simulink model "ES2_4_simulink"  (R2023b)
settings: Solver=VariableStepAuto  StartTime=0.0  StopTime=30.0  RelTol=1e-3
undefined symbols (not defined in the file): fdesignblkfcn, gcbh
libraries: dspfdesign x4, dspstat3 x4, simulink x4, vrlib x2
settings Model: NumberOfSteps=100  Creator=manu  LastModifiedBy=manu

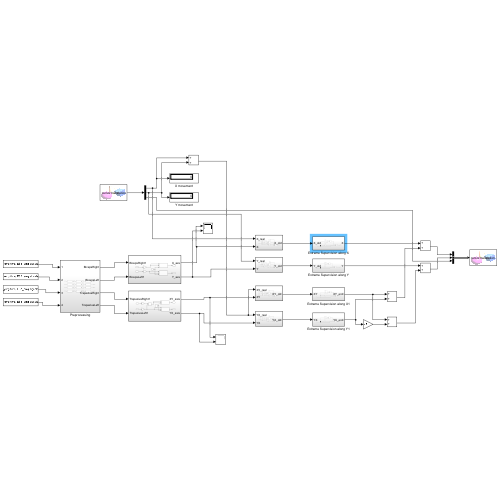
[thumbnail: Simulink's stored preview of the top-level diagram]
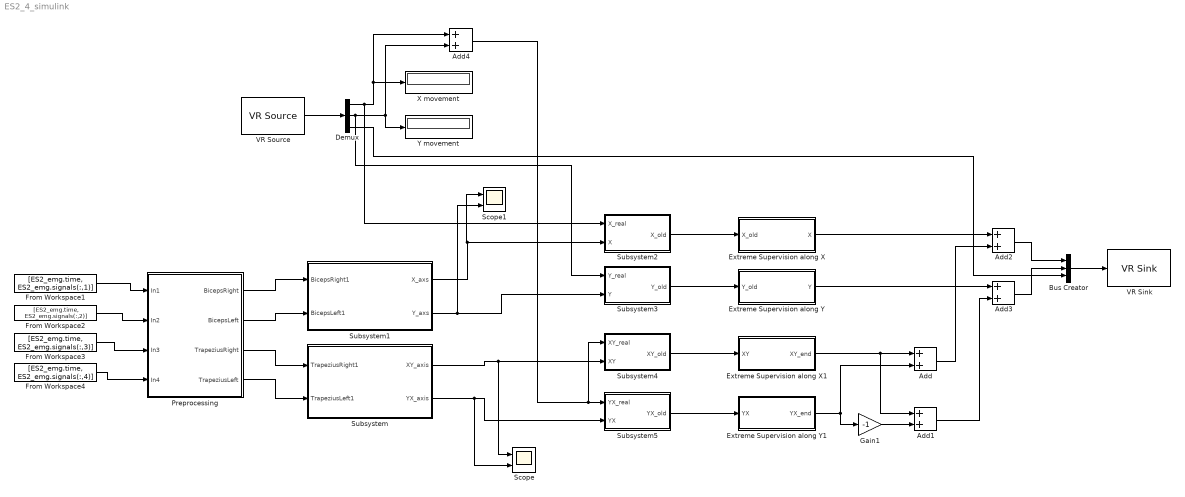
== system ES2_4_simulink ==
  Add{,1..4} (5 alike) : Sum
  Bus Creator : BusCreator  Inputs=3
  Demux : Demux  Outputs=3
  Extreme Supervision along X : Subsystem
  Extreme Supervision along X1 : Subsystem
  Extreme Supervision along Y : Subsystem
  Extreme Supervision along Y1 : Subsystem
  From Workspace1 : FromWorkspace  VariableName=[ES2_emg.time, ES2_emg.signals(:,1)]  OutDataTypeStr=double  SampleTime=0.001
  From Workspace2 : FromWorkspace  VariableName=[ES2_emg.time, ES2_emg.signals(:,2)]  OutDataTypeStr=double  SampleTime=0.001
  From Workspace3 : FromWorkspace  VariableName=[ES2_emg.time, ES2_emg.signals(:,3)]  OutDataTypeStr=double  SampleTime=0.001
  From Workspace4 : FromWorkspace  VariableName=[ES2_emg.time, ES2_emg.signals(:,4)]  OutDataTypeStr=double  SampleTime=0.001
  Gain1 : Gain  Gain=-1
  Preprocessing : Subsystem
  Scope : Scope  NumInputPorts=2
  Scope1 : Scope  NumInputPorts=2
  Subsystem : Subsystem
  Subsystem1 : Subsystem
  Subsystem2 : Subsystem
  Subsystem3 : Subsystem
  Subsystem4 : Subsystem
  Subsystem5 : Subsystem
  VR Sink : vrlib/VR Sink  InstantiateOnLoad=on  SampleTime=0.1  ViewEnable=on  RemoteChange=off  RemoteView=off  FieldsWritten=cursor.translation.3.1.1.double  WorldFileName=8_palline_color.wrl  AutoView=off  VideoDimensions=[]  AllowVariableSize=off
  VR Source : vrlib/VR Source  InstantiateOnLoad=on  SampleTime=0.1  ViewEnable=on  RemoteChange=off  RemoteView=off  FieldsRead=cursor.translation.1.3.1.double  WorldFileName=8_palline_color.wrl  AutoView=off  VideoDimensions=[]  AllowVariableSize=off
  X movement : Display
  Y movement : Display
  wires:
  From Workspace1/1 -> Preprocessing/1(In1)
  From Workspace2/1 -> Preprocessing/2(In2)
  From Workspace3/1 -> Preprocessing/3(In3)
  From Workspace4/1 -> Preprocessing/4(In4)
  Bus Creator/1 -> VR Sink/1
  VR Source/1 -> Demux/1
  Demux/3 -> Bus Creator/3
  Demux/1 -> Subsystem2/1(X_real), X movement/1, Add4/1
  Demux/2 -> Y movement/1, Add4/2, Subsystem3/1(Y_real)
  Subsystem1/1(X_axs) -> Scope1/1, Subsystem2/2(X)
  Subsystem2/1(X_old) -> Extreme Supervision along X/1(X_old)
  Subsystem1/2(Y_axs) -> Scope1/2, Subsystem3/2(Y)
  Subsystem3/1(Y_old) -> Extreme Supervision along Y/1(Y_old)
  Add/1 -> Add2/2
  Extreme Supervision along X1/1(XY_end) -> Add1/1, Add/1
  Extreme Supervision along Y1/1(YX_end) -> Gain1/1, Add/2
  Gain1/1 -> Add1/2
  Add1/1 -> Add3/2
  Extreme Supervision along X/1(X) -> Add2/1
  Add2/1 -> Bus Creator/1
  Extreme Supervision along Y/1(Y) -> Add3/1
  Add3/1 -> Bus Creator/2
  Subsystem4/1(XY_old) -> Extreme Supervision along X1/1(XY)
  Subsystem5/1(YX_old) -> Extreme Supervision along Y1/1(YX)
  Add4/1 -> Subsystem5/1(YX_real), Subsystem4/1(XY_real)
  Preprocessing/1(BicepsRight) -> Subsystem1/1(BicepsRight1)
  Preprocessing/2(BicepsLeft) -> Subsystem1/2(BicepsLeft1)
  Preprocessing/3(TrapeziusRight) -> Subsystem/1(TrapeziusRight1)
  Preprocessing/4(TrapeziusLeft) -> Subsystem/2(TrapeziusLeft1)
  Subsystem/1(XY_axis) -> Subsystem4/2(XY), Scope/1
  Subsystem/2(YX_axis) -> Scope/2, Subsystem5/2(YX)

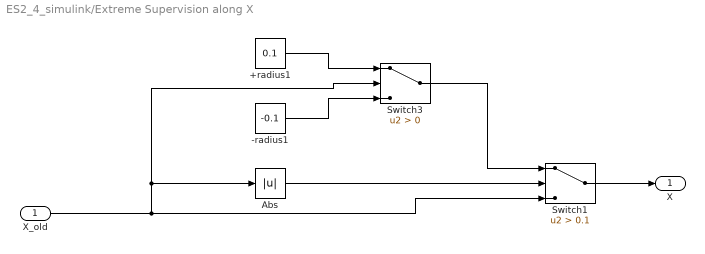
== system ES2_4_simulink/Extreme Supervision along X ==
  X_old : Inport
  +radius1 : Constant  Value=0.1
  -radius1 : Constant  Value=-0.1
  Abs : Abs  SaturateOnIntegerOverflow=off
  Switch1 : Switch  Criteria=u2 > Threshold  Threshold=0.1  SaturateOnIntegerOverflow=off  InputSameDT=off
  Switch3 : Switch  Criteria=u2 > Threshold  SaturateOnIntegerOverflow=off  InputSameDT=off
  X : Outport
  wires:
  Switch3/1 -> Switch1/1
  Abs/1 -> Switch1/2
  +radius1/1 -> Switch3/1
  X_old/1 -> Switch3/2, Abs/1, Switch1/3
  -radius1/1 -> Switch3/3
  Switch1/1 -> X/1

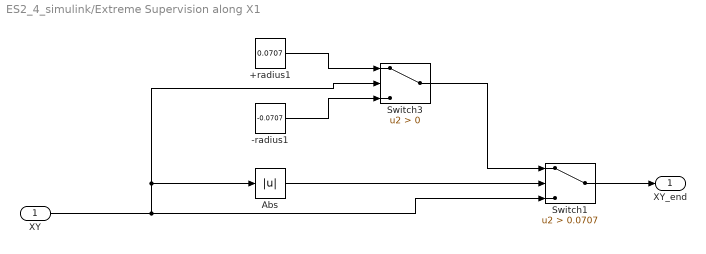
== system ES2_4_simulink/Extreme Supervision along X1 ==
  XY : Inport
  +radius1 : Constant  Value=0.0707
  -radius1 : Constant  Value=-0.0707
  Abs : Abs  SaturateOnIntegerOverflow=off
  Switch1 : Switch  Criteria=u2 > Threshold  Threshold=0.0707  SaturateOnIntegerOverflow=off  InputSameDT=off
  Switch3 : Switch  Criteria=u2 > Threshold  SaturateOnIntegerOverflow=off  InputSameDT=off
  XY_end : Outport
  wires:
  Switch3/1 -> Switch1/1
  Abs/1 -> Switch1/2
  +radius1/1 -> Switch3/1
  XY/1 -> Switch3/2, Abs/1, Switch1/3
  -radius1/1 -> Switch3/3
  Switch1/1 -> XY_end/1

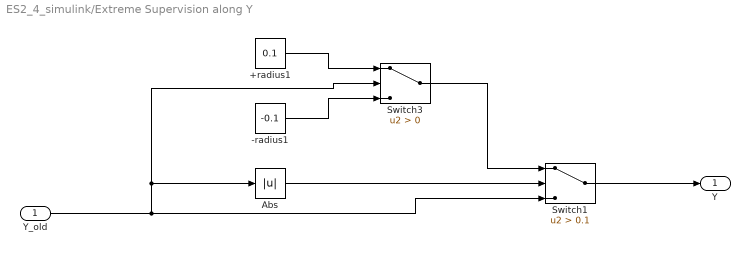
== system ES2_4_simulink/Extreme Supervision along Y ==
  Y_old : Inport
  +radius1 : Constant  Value=0.1
  -radius1 : Constant  Value=-0.1
  Abs : Abs  SaturateOnIntegerOverflow=off
  Switch1 : Switch  Criteria=u2 > Threshold  Threshold=0.1  SaturateOnIntegerOverflow=off  InputSameDT=off
  Switch3 : Switch  Criteria=u2 > Threshold  SaturateOnIntegerOverflow=off  InputSameDT=off
  Y : Outport
  wires:
  Switch3/1 -> Switch1/1
  Abs/1 -> Switch1/2
  +radius1/1 -> Switch3/1
  Y_old/1 -> Switch3/2, Abs/1, Switch1/3
  -radius1/1 -> Switch3/3
  Switch1/1 -> Y/1

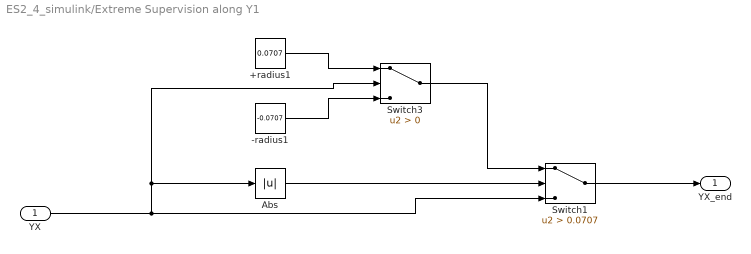
== system ES2_4_simulink/Extreme Supervision along Y1 ==
  YX : Inport
  +radius1 : Constant  Value=0.0707
  -radius1 : Constant  Value=-0.0707
  Abs : Abs  SaturateOnIntegerOverflow=off
  Switch1 : Switch  Criteria=u2 > Threshold  Threshold=0.0707  SaturateOnIntegerOverflow=off  InputSameDT=off
  Switch3 : Switch  Criteria=u2 > Threshold  SaturateOnIntegerOverflow=off  InputSameDT=off
  YX_end : Outport
  wires:
  Switch3/1 -> Switch1/1
  Abs/1 -> Switch1/2
  +radius1/1 -> Switch3/1
  YX/1 -> Switch3/2, Abs/1, Switch1/3
  -radius1/1 -> Switch3/3
  Switch1/1 -> YX_end/1

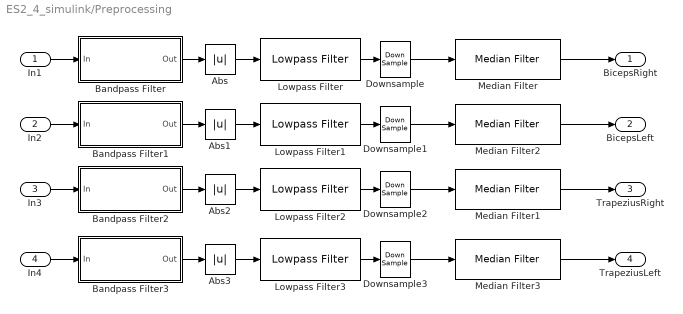
== system ES2_4_simulink/Preprocessing ==
  In1 : Inport
  In2 : Inport  Port=2
  In3 : Inport  Port=3
  In4 : Inport  Port=4
  Abs{,1..3} (4 alike) : Abs  SaturateOnIntegerOverflow=off
  Bandpass Filter : Subsystem  DialogController=fdesignblkfcn  InitFcn=fdesignblkfcn(gcbh, {'InitFcn'});  mask(Bandpass Filter){}
      mask help: dsp:DSPFilterDesignBlockDialog:BandpassFdesign_MaskDesc
      settings: CopyFcn=fdesignblkfcn(gcbh, {'CopyFcn'});
      mask Help: helpview(mapfilelocation('dsp'), 'dspbandpassfilter');
      mask Display: disp('Bandpass');
  Bandpass Filter1 : Subsystem  DialogController=fdesignblkfcn  InitFcn=fdesignblkfcn(gcbh, {'InitFcn'});  mask(Bandpass Filter){}
      mask help: dsp:DSPFilterDesignBlockDialog:BandpassFdesign_MaskDesc
      settings: CopyFcn=fdesignblkfcn(gcbh, {'CopyFcn'});
      mask Help: helpview(mapfilelocation('dsp'), 'dspbandpassfilter');
      mask Display: disp('Bandpass');
  Bandpass Filter2 : Subsystem  DialogController=fdesignblkfcn  InitFcn=fdesignblkfcn(gcbh, {'InitFcn'});  mask(Bandpass Filter){}
      mask help: dsp:DSPFilterDesignBlockDialog:BandpassFdesign_MaskDesc
      settings: CopyFcn=fdesignblkfcn(gcbh, {'CopyFcn'});
      mask Help: helpview(mapfilelocation('dsp'), 'dspbandpassfilter');
      mask Display: disp('Bandpass');
  Bandpass Filter3 : Subsystem  DialogController=fdesignblkfcn  InitFcn=fdesignblkfcn(gcbh, {'InitFcn'});  mask(Bandpass Filter){}
      mask help: dsp:DSPFilterDesignBlockDialog:BandpassFdesign_MaskDesc
      settings: CopyFcn=fdesignblkfcn(gcbh, {'CopyFcn'});
      mask Help: helpview(mapfilelocation('dsp'), 'dspbandpassfilter');
      mask Display: disp('Bandpass');
  Downsample{,1..3} (4 alike) : DownSample  N=4  RateOptions=Allow multirate processing
  Lowpass Filter{,1..3} (4 alike) : dspfdesign/Lowpass Filter  FilterType=FIR  DesignForMinimumOrder=on  FilterOrder=50  PassbandFrequency=3  StopbandFrequency=6  PassbandRipple=0.1  StopbandAttenuation=80  SampleRateMode=Specify on dialog  SampleRate=1000  SimulateUsing=Interpreted execution  roundingMode=Floor  coeffsDataTypeStr=fixdt(1,16)
  Median Filter : dspstat3/Median Filter  WindowLength=250  SimulateUsing=Interpreted execution
      settings: LibrarySourceBlock=|
      | dspfdesign/Median
      | Filter
  Median Filter1 : dspstat3/Median Filter  WindowLength=300  SimulateUsing=Interpreted execution
      settings: LibrarySourceBlock=|
      | dspfdesign/Median
      | Filter
  Median Filter2 : dspstat3/Median Filter  WindowLength=250  SimulateUsing=Interpreted execution
      settings: LibrarySourceBlock=|
      | dspfdesign/Median
      | Filter
  Median Filter3 : dspstat3/Median Filter  WindowLength=250  SimulateUsing=Interpreted execution
      settings: LibrarySourceBlock=|
      | dspfdesign/Median
      | Filter
  BicepsRight : Outport
  BicepsLeft : Outport  Port=2
  TrapeziusRight : Outport  Port=3
  TrapeziusLeft : Outport  Port=4
  wires:
  Lowpass Filter2/1 -> Downsample2/1
  Bandpass Filter2/1(Out) -> Abs2/1
  Abs1/1 -> Lowpass Filter1/1
  Abs3/1 -> Lowpass Filter3/1
  Abs/1 -> Lowpass Filter/1
  Bandpass Filter3/1(Out) -> Abs3/1
  In4/1 -> Bandpass Filter3/1(In)
  In1/1 -> Bandpass Filter/1(In)
  Bandpass Filter/1(Out) -> Abs/1
  Bandpass Filter1/1(Out) -> Abs1/1
  Abs2/1 -> Lowpass Filter2/1
  Lowpass Filter1/1 -> Downsample1/1
  Lowpass Filter3/1 -> Downsample3/1
  Lowpass Filter/1 -> Downsample/1
  In3/1 -> Bandpass Filter2/1(In)
  In2/1 -> Bandpass Filter1/1(In)
  Downsample/1 -> Median Filter/1
  Downsample1/1 -> Median Filter2/1
  Downsample2/1 -> Median Filter1/1
  Downsample3/1 -> Median Filter3/1
  Median Filter/1 -> BicepsRight/1
  Median Filter2/1 -> BicepsLeft/1
  Median Filter1/1 -> TrapeziusRight/1
  Median Filter3/1 -> TrapeziusLeft/1

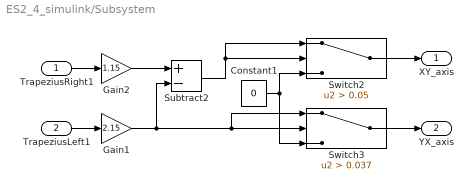
== system ES2_4_simulink/Subsystem ==
  TrapeziusRight1 : Inport
  TrapeziusLeft1 : Inport  Port=2
  Constant1 : Constant  Value=0
  Gain1 : Gain  Gain=2.15
  Gain2 : Gain  Gain=1.15
  Subtract2 : Sum  Inputs=+-
  Switch2 : Switch  Criteria=u2 > Threshold  Threshold=0.05  SaturateOnIntegerOverflow=off  InputSameDT=off
  Switch3 : Switch  Criteria=u2 > Threshold  Threshold=0.037  SaturateOnIntegerOverflow=off  InputSameDT=off
  XY_axis : Outport
  YX_axis : Outport  Port=2
  wires:
  TrapeziusRight1/1 -> Gain2/1
  Constant1/1 -> Switch3/3, Switch2/3
  Gain1/1 -> Subtract2/2, Switch3/1, Switch3/2
  Gain2/1 -> Subtract2/1
  TrapeziusLeft1/1 -> Gain1/1
  Subtract2/1 -> Switch2/1, Switch2/2
  Switch2/1 -> XY_axis/1
  Switch3/1 -> YX_axis/1

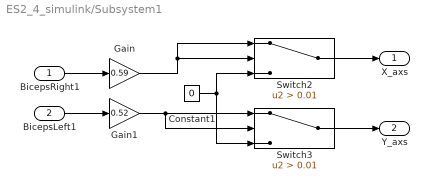
== system ES2_4_simulink/Subsystem1 ==
  BicepsRight1 : Inport
  BicepsLeft1 : Inport  Port=2
  Constant1 : Constant  Value=0
  Gain : Gain  Gain=0.59
  Gain1 : Gain  Gain=0.52
  Switch2 : Switch  Criteria=u2 > Threshold  Threshold=0.01  SaturateOnIntegerOverflow=off  InputSameDT=off
  Switch3 : Switch  Criteria=u2 > Threshold  Threshold=0.01  SaturateOnIntegerOverflow=off  InputSameDT=off
  X_axs : Outport
  Y_axs : Outport  Port=2
  wires:
  BicepsLeft1/1 -> Gain1/1
  BicepsRight1/1 -> Gain/1
  Constant1/1 -> Switch3/3, Switch2/3
  Gain/1 -> Switch2/1, Switch2/2
  Gain1/1 -> Switch3/1, Switch3/2
  Switch2/1 -> X_axs/1
  Switch3/1 -> Y_axs/1

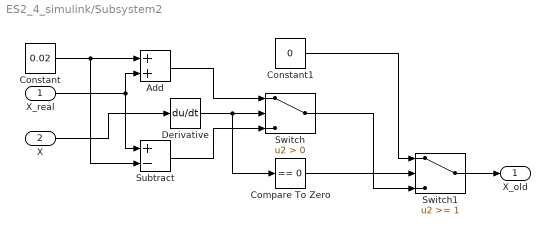
== system ES2_4_simulink/Subsystem2 ==
  X_real : Inport
  X : Inport  Port=2
  Add : Sum
  Compare To Zero : simulink/Logic and Bit Operations/Compare To Zero  relop===  OutDataTypeStr=boolean
  Constant : Constant  Value=0.02
  Constant1 : Constant  Value=0
  Derivative : Derivative
  Subtract : Sum  Inputs=+-
  Switch : Switch  Criteria=u2 > Threshold  SaturateOnIntegerOverflow=off  InputSameDT=off
  Switch1 : Switch  Threshold=1  SaturateOnIntegerOverflow=off  InputSameDT=off
  X_old : Outport
  wires:
  Derivative/1 -> Compare To Zero/1, Switch/2
  Compare To Zero/1 -> Switch1/2
  Constant/1 -> Add/1, Subtract/2
  X_real/1 -> Subtract/1, Add/2
  Constant1/1 -> Switch1/1
  Switch/1 -> Switch1/3
  Add/1 -> Switch/1
  Subtract/1 -> Switch/3
  X/1 -> Derivative/1
  Switch1/1 -> X_old/1

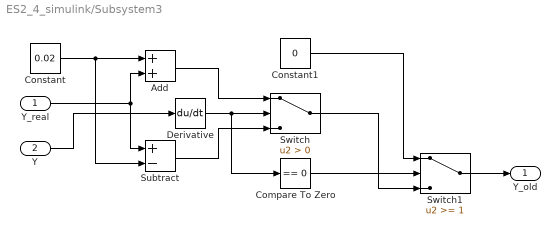
== system ES2_4_simulink/Subsystem3 ==
  Y_real : Inport
  Y : Inport  Port=2
  Add : Sum
  Compare To Zero : simulink/Logic and Bit Operations/Compare To Zero  relop===  OutDataTypeStr=boolean
  Constant : Constant  Value=0.02
  Constant1 : Constant  Value=0
  Derivative : Derivative
  Subtract : Sum  Inputs=+-
  Switch : Switch  Criteria=u2 > Threshold  SaturateOnIntegerOverflow=off  InputSameDT=off
  Switch1 : Switch  Threshold=1  SaturateOnIntegerOverflow=off  InputSameDT=off
  Y_old : Outport
  wires:
  Derivative/1 -> Compare To Zero/1, Switch/2
  Compare To Zero/1 -> Switch1/2
  Constant/1 -> Add/1, Subtract/2
  Y_real/1 -> Add/2, Subtract/1
  Constant1/1 -> Switch1/1
  Switch/1 -> Switch1/3
  Add/1 -> Switch/1
  Subtract/1 -> Switch/3
  Y/1 -> Derivative/1
  Switch1/1 -> Y_old/1

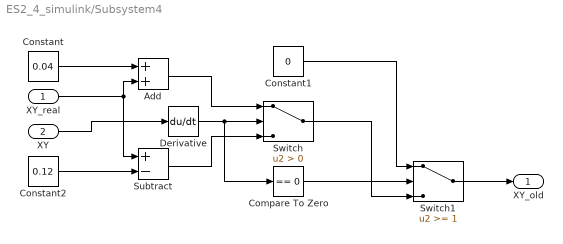
== system ES2_4_simulink/Subsystem4 ==
  XY_real : Inport
  XY : Inport  Port=2
  Add : Sum
  Compare To Zero : simulink/Logic and Bit Operations/Compare To Zero  relop===  OutDataTypeStr=boolean
  Constant : Constant  Value=0.04
  Constant1 : Constant  Value=0
  Constant2 : Constant  Value=0.12
  Derivative : Derivative
  Subtract : Sum  Inputs=+-
  Switch : Switch  Criteria=u2 > Threshold  SaturateOnIntegerOverflow=off  InputSameDT=off
  Switch1 : Switch  Threshold=1  SaturateOnIntegerOverflow=off  InputSameDT=off
  XY_old : Outport
  wires:
  Derivative/1 -> Compare To Zero/1, Switch/2
  Compare To Zero/1 -> Switch1/2
  Constant/1 -> Add/1
  XY_real/1 -> Add/2, Subtract/1
  Constant1/1 -> Switch1/1
  Switch/1 -> Switch1/3
  Add/1 -> Switch/1
  Subtract/1 -> Switch/3
  XY/1 -> Derivative/1
  Switch1/1 -> XY_old/1
  Constant2/1 -> Subtract/2

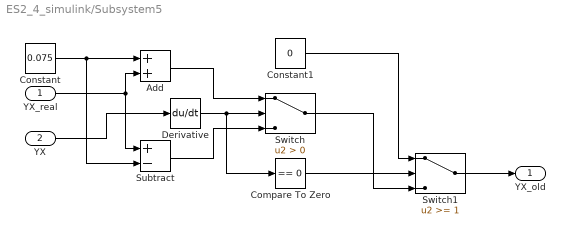
== system ES2_4_simulink/Subsystem5 ==
  YX_real : Inport
  YX : Inport  Port=2
  Add : Sum
  Compare To Zero : simulink/Logic and Bit Operations/Compare To Zero  relop===  OutDataTypeStr=boolean
  Constant : Constant  Value=0.075
  Constant1 : Constant  Value=0
  Derivative : Derivative
  Subtract : Sum  Inputs=+-
  Switch : Switch  Criteria=u2 > Threshold  SaturateOnIntegerOverflow=off  InputSameDT=off
  Switch1 : Switch  Threshold=1  SaturateOnIntegerOverflow=off  InputSameDT=off
  YX_old : Outport
  wires:
  Derivative/1 -> Compare To Zero/1, Switch/2
  Compare To Zero/1 -> Switch1/2
  Constant/1 -> Subtract/2, Add/1
  YX_real/1 -> Subtract/1, Add/2
  Constant1/1 -> Switch1/1
  Switch/1 -> Switch1/3
  Add/1 -> Switch/1
  Subtract/1 -> Switch/3
  YX/1 -> Derivative/1
  Switch1/1 -> YX_old/1

== system ES2_4_simulink/Preprocessing/Bandpass Filter ==
  In : Inport
  Generated Filter Block : DiscreteFir  Tag=BlockMethodSubSystem  Coefficients=[8.09984662039171167e-19 6.39138873735445952e-05 -0.000529985360713195602 0.000163049509978640958 -0.00106873656065133355 0.000138454107623771778 -0.00150740219393306354 -0.000146171169312381939 -0.00164491285071874664 -0.000803831165663842096 -0.00127002939103642264 -0.00179475969145176406 -0.000313202715390952153 -0.00280047053638836797 0.00102378750565708626 -0.00320898606072516192 0.00226847122552957785 -0.00229118992766688115 0.00286273128519679053 0.000444283590646493102 0.00248061645378650983 0.00484772649949967091 0.0013231555973298554 0.00988516690279817554 0.000195375038696813459 0.0137475146561206515 0.000235578061564314939 0.0143783789118079978 0.00232373851233996093 0.0102932854869860792 0.00637980828249819481 0.0013872101835551594 0.0108821641584975915 -0.0106388069047137126 0.0129164407258158982 -0.0225052497171089536 0.00888838159476280226 -0.0302697542973048087 -0.00424164083303872359 -0.0306714306083059364 -0.0276065409272709811 -0.022423923961180349 -0.0594922495550082378 -0.00693651358874992994 -0.0952531612511480497 0.0118816213758879876 -0.128243809353299015 0.0287429432612043914 -0.151547652016043505 0.0386729267839347052 0.839787881504184819 0.0386729267839347052 -0.151547652016043505 0.0287429432612043914 -0.128243809353299015 0.0118816213758879876 -0.0952531612511480497 -0.00693651358874992994 -0.0594922495550082378 -0.022423923961180349 -0.0276065409272709811 -0.0306714306083059364 -0.00424164083303872359 -0.0302697542973048087 0.00888838159476280226 -0.0225052497171089536 0.0129164407258158982 -0.0106388069047137126 0.0108821641584975915 0.0013872101835551594 0.00637980828249819481 0.0102932854869860792 0.00232373851233996093 0.0143783789118079978 0.000235578061564314939 0.0137475146561206515 0.000195375038696813459 0.00988516690279817554 0.0013231555973298554 0.00484772649949967091 0.00248061645378650983 0.000444283590646493102 0.00286273128519679053 -0.00229118992766688115 0.00226847122552957785 -0.00320898606072516192 0.00102378750565708626 -0.00280047053638836797 -0.000313202715390952153 -0.00179475969145176406 -0.00127002939103642264 -0.000803831165663842096 -0.00164491285071874664 -0.000146171169312381939 -0.00150740219393306354 0.000138454107623771778 -0.00106873656065133355 0.000163049509978640958 -0.000529985360713195602 6.39138873735445952e-05 8.09984662039171167e-19]  InputProcessing=Columns as channels (frame based)
  Out : Outport  VectorParamsAs1DForOutWhenUnconnected=off
  wires:
  In/1 -> Generated Filter Block/1
  Generated Filter Block/1 -> Out/1

== system ES2_4_simulink/Preprocessing/Bandpass Filter1 ==
  In : Inport
  Generated Filter Block : DiscreteFir  Tag=BlockMethodSubSystem  Coefficients=[8.09984662039171167e-19 6.39138873735445952e-05 -0.000529985360713195602 0.000163049509978640958 -0.00106873656065133355 0.000138454107623771778 -0.00150740219393306354 -0.000146171169312381939 -0.00164491285071874664 -0.000803831165663842096 -0.00127002939103642264 -0.00179475969145176406 -0.000313202715390952153 -0.00280047053638836797 0.00102378750565708626 -0.00320898606072516192 0.00226847122552957785 -0.00229118992766688115 0.00286273128519679053 0.000444283590646493102 0.00248061645378650983 0.00484772649949967091 0.0013231555973298554 0.00988516690279817554 0.000195375038696813459 0.0137475146561206515 0.000235578061564314939 0.0143783789118079978 0.00232373851233996093 0.0102932854869860792 0.00637980828249819481 0.0013872101835551594 0.0108821641584975915 -0.0106388069047137126 0.0129164407258158982 -0.0225052497171089536 0.00888838159476280226 -0.0302697542973048087 -0.00424164083303872359 -0.0306714306083059364 -0.0276065409272709811 -0.022423923961180349 -0.0594922495550082378 -0.00693651358874992994 -0.0952531612511480497 0.0118816213758879876 -0.128243809353299015 0.0287429432612043914 -0.151547652016043505 0.0386729267839347052 0.839787881504184819 0.0386729267839347052 -0.151547652016043505 0.0287429432612043914 -0.128243809353299015 0.0118816213758879876 -0.0952531612511480497 -0.00693651358874992994 -0.0594922495550082378 -0.022423923961180349 -0.0276065409272709811 -0.0306714306083059364 -0.00424164083303872359 -0.0302697542973048087 0.00888838159476280226 -0.0225052497171089536 0.0129164407258158982 -0.0106388069047137126 0.0108821641584975915 0.0013872101835551594 0.00637980828249819481 0.0102932854869860792 0.00232373851233996093 0.0143783789118079978 0.000235578061564314939 0.0137475146561206515 0.000195375038696813459 0.00988516690279817554 0.0013231555973298554 0.00484772649949967091 0.00248061645378650983 0.000444283590646493102 0.00286273128519679053 -0.00229118992766688115 0.00226847122552957785 -0.00320898606072516192 0.00102378750565708626 -0.00280047053638836797 -0.000313202715390952153 -0.00179475969145176406 -0.00127002939103642264 -0.000803831165663842096 -0.00164491285071874664 -0.000146171169312381939 -0.00150740219393306354 0.000138454107623771778 -0.00106873656065133355 0.000163049509978640958 -0.000529985360713195602 6.39138873735445952e-05 8.09984662039171167e-19]  InputProcessing=Columns as channels (frame based)
  Out : Outport  VectorParamsAs1DForOutWhenUnconnected=off
  wires:
  In/1 -> Generated Filter Block/1
  Generated Filter Block/1 -> Out/1

== system ES2_4_simulink/Preprocessing/Bandpass Filter2 ==
  In : Inport
  Generated Filter Block : DiscreteFir  Tag=BlockMethodSubSystem  Coefficients=[8.09984662039171167e-19 6.39138873735445952e-05 -0.000529985360713195602 0.000163049509978640958 -0.00106873656065133355 0.000138454107623771778 -0.00150740219393306354 -0.000146171169312381939 -0.00164491285071874664 -0.000803831165663842096 -0.00127002939103642264 -0.00179475969145176406 -0.000313202715390952153 -0.00280047053638836797 0.00102378750565708626 -0.00320898606072516192 0.00226847122552957785 -0.00229118992766688115 0.00286273128519679053 0.000444283590646493102 0.00248061645378650983 0.00484772649949967091 0.0013231555973298554 0.00988516690279817554 0.000195375038696813459 0.0137475146561206515 0.000235578061564314939 0.0143783789118079978 0.00232373851233996093 0.0102932854869860792 0.00637980828249819481 0.0013872101835551594 0.0108821641584975915 -0.0106388069047137126 0.0129164407258158982 -0.0225052497171089536 0.00888838159476280226 -0.0302697542973048087 -0.00424164083303872359 -0.0306714306083059364 -0.0276065409272709811 -0.022423923961180349 -0.0594922495550082378 -0.00693651358874992994 -0.0952531612511480497 0.0118816213758879876 -0.128243809353299015 0.0287429432612043914 -0.151547652016043505 0.0386729267839347052 0.839787881504184819 0.0386729267839347052 -0.151547652016043505 0.0287429432612043914 -0.128243809353299015 0.0118816213758879876 -0.0952531612511480497 -0.00693651358874992994 -0.0594922495550082378 -0.022423923961180349 -0.0276065409272709811 -0.0306714306083059364 -0.00424164083303872359 -0.0302697542973048087 0.00888838159476280226 -0.0225052497171089536 0.0129164407258158982 -0.0106388069047137126 0.0108821641584975915 0.0013872101835551594 0.00637980828249819481 0.0102932854869860792 0.00232373851233996093 0.0143783789118079978 0.000235578061564314939 0.0137475146561206515 0.000195375038696813459 0.00988516690279817554 0.0013231555973298554 0.00484772649949967091 0.00248061645378650983 0.000444283590646493102 0.00286273128519679053 -0.00229118992766688115 0.00226847122552957785 -0.00320898606072516192 0.00102378750565708626 -0.00280047053638836797 -0.000313202715390952153 -0.00179475969145176406 -0.00127002939103642264 -0.000803831165663842096 -0.00164491285071874664 -0.000146171169312381939 -0.00150740219393306354 0.000138454107623771778 -0.00106873656065133355 0.000163049509978640958 -0.000529985360713195602 6.39138873735445952e-05 8.09984662039171167e-19]  InputProcessing=Columns as channels (frame based)
  Out : Outport  VectorParamsAs1DForOutWhenUnconnected=off
  wires:
  In/1 -> Generated Filter Block/1
  Generated Filter Block/1 -> Out/1

== system ES2_4_simulink/Preprocessing/Bandpass Filter3 ==
  In : Inport
  Generated Filter Block : DiscreteFir  Tag=BlockMethodSubSystem  Coefficients=[8.09984662039171167e-19 6.39138873735445952e-05 -0.000529985360713195602 0.000163049509978640958 -0.00106873656065133355 0.000138454107623771778 -0.00150740219393306354 -0.000146171169312381939 -0.00164491285071874664 -0.000803831165663842096 -0.00127002939103642264 -0.00179475969145176406 -0.000313202715390952153 -0.00280047053638836797 0.00102378750565708626 -0.00320898606072516192 0.00226847122552957785 -0.00229118992766688115 0.00286273128519679053 0.000444283590646493102 0.00248061645378650983 0.00484772649949967091 0.0013231555973298554 0.00988516690279817554 0.000195375038696813459 0.0137475146561206515 0.000235578061564314939 0.0143783789118079978 0.00232373851233996093 0.0102932854869860792 0.00637980828249819481 0.0013872101835551594 0.0108821641584975915 -0.0106388069047137126 0.0129164407258158982 -0.0225052497171089536 0.00888838159476280226 -0.0302697542973048087 -0.00424164083303872359 -0.0306714306083059364 -0.0276065409272709811 -0.022423923961180349 -0.0594922495550082378 -0.00693651358874992994 -0.0952531612511480497 0.0118816213758879876 -0.128243809353299015 0.0287429432612043914 -0.151547652016043505 0.0386729267839347052 0.839787881504184819 0.0386729267839347052 -0.151547652016043505 0.0287429432612043914 -0.128243809353299015 0.0118816213758879876 -0.0952531612511480497 -0.00693651358874992994 -0.0594922495550082378 -0.022423923961180349 -0.0276065409272709811 -0.0306714306083059364 -0.00424164083303872359 -0.0302697542973048087 0.00888838159476280226 -0.0225052497171089536 0.0129164407258158982 -0.0106388069047137126 0.0108821641584975915 0.0013872101835551594 0.00637980828249819481 0.0102932854869860792 0.00232373851233996093 0.0143783789118079978 0.000235578061564314939 0.0137475146561206515 0.000195375038696813459 0.00988516690279817554 0.0013231555973298554 0.00484772649949967091 0.00248061645378650983 0.000444283590646493102 0.00286273128519679053 -0.00229118992766688115 0.00226847122552957785 -0.00320898606072516192 0.00102378750565708626 -0.00280047053638836797 -0.000313202715390952153 -0.00179475969145176406 -0.00127002939103642264 -0.000803831165663842096 -0.00164491285071874664 -0.000146171169312381939 -0.00150740219393306354 0.000138454107623771778 -0.00106873656065133355 0.000163049509978640958 -0.000529985360713195602 6.39138873735445952e-05 8.09984662039171167e-19]  InputProcessing=Columns as channels (frame based)
  Out : Outport  VectorParamsAs1DForOutWhenUnconnected=off
  wires:
  In/1 -> Generated Filter Block/1
  Generated Filter Block/1 -> Out/1
